simulink model "ThreeFeeder"  (R2023b)
settings: Solver=FixedStepDiscrete  StartTime=0.0  StopTime=2  RelTol=1e-3
InitFcn:
  | Frequency = 50;
  | w = 2*pi*Frequency;
  | 
  | Vnom_ph_ph = 22000;
  | Vnom = Vnom_ph_ph/sqrt(3);
  | 
  | % miles/km
  | mi2km = 1.60934;
  | % feet to km
  | ft2km = 0.0003048;
  | % microsiemens to Farads
  | ms2F = 1/2/pi/60*1e-6;
  | 
  | % Breaker
  | NOP1 = 0;
  | NOP2 = 0;
  | NOP3 = 0;
  | Fault = 0;
  | CB1 = 1;
  | CB2 = 1;
  | CB3 = 1;
undefined symbols (not defined in the file): Angle, D11, Delta, Magnitude
libraries: spsLoadFlowBusLib x24, spsThreePhasePISectionLineLib x22, spsThreePhaseVIMeasurementLib x21, spsThreePhaseSeriesRLCLoadLib x18, spsCurrentMeasurementLib x9, spsGroundLib x9, spsVoltageMeasurementLib x9, spsThreePhaseBreakerLib x6, spsThreePhaseSeriesRLCBranchLib x6, spsThreePhaseSourceLib x4, spsThreePhaseTransformerTwoWindingsLib x3, spsThreePhaseFaultLib x1
(part 1 of 2)
settings Model: Creator=liyifu  LastModifiedBy=liyifu
settings SolverCC: AlgebraicLoopSolver=TrustRegion
settings DataIOCC: ReturnWorkspaceOutputs=off
settings OptimizationCC: ReuseModelBlockBuffer=off
settings DebuggingCC: UnconnectedInputMsg=warning  UnconnectedOutputMsg=warning  UnconnectedLineMsg=warning  ArithmeticOperatorsInVariantConditions=warning
settings ModelReferenceCC: EnableRefExpFcnMdlSchedulingChecks=on
settings SFSimCC: SimUseLocalCustomCode=off  CustomCodeUndefinedFunction=UseInterfaceOnly
settings RTWCC: RTWUseLocalCustomCode=off

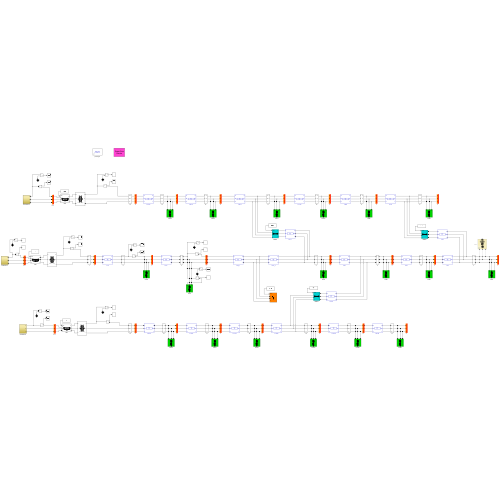
[thumbnail: Simulink's stored preview of the top-level diagram]
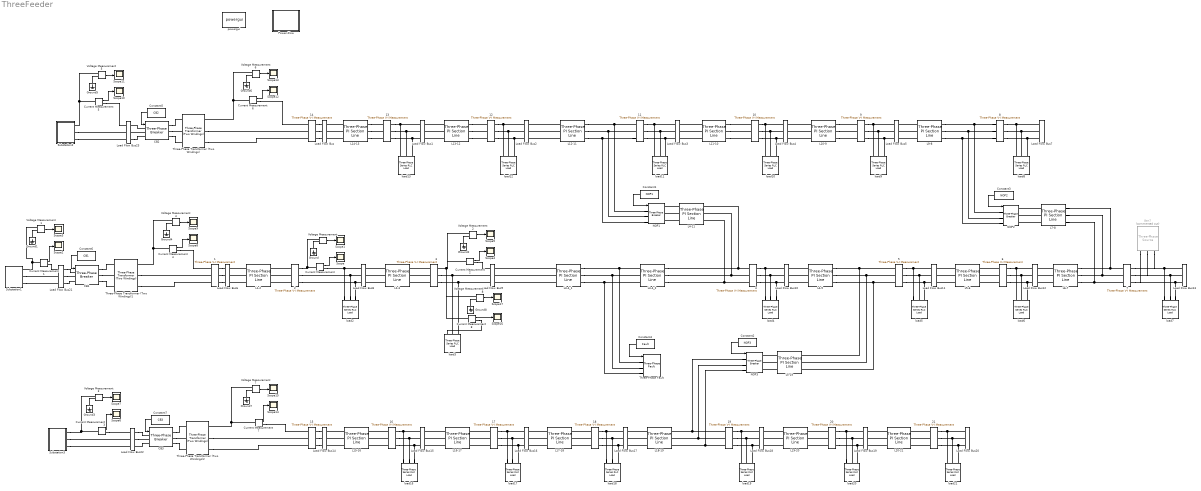
== system ThreeFeeder ==
  1 : spsThreePhaseVIMeasurementLib/Three-Phase V-I Measurement  VoltageMeasurement=phase-to-ground  SetLabelV=on  LabelV=Vabc_1  Vpu=on  VpuLL=off  CurrentMeasurement=yes  SetLabelI=on  LabelI=Iabc_1  Ipu=on  Pbase=100e6  Vbase=Vnom_ph_ph  OutputType=Magnitude-Angle  PhasorSimulation=off  PSBequivalent=0
  10 : spsThreePhaseVIMeasurementLib/Three-Phase V-I Measurement  VoltageMeasurement=phase-to-ground  SetLabelV=on  LabelV=Vabc_10  Vpu=on  VpuLL=off  CurrentMeasurement=yes  SetLabelI=on  LabelI=Iabc_10  Ipu=on  Pbase=100e6  Vbase=Vnom_ph_ph  OutputType=Magnitude-Angle  PhasorSimulation=off  PSBequivalent=0
  11 : spsThreePhaseVIMeasurementLib/Three-Phase V-I Measurement  VoltageMeasurement=phase-to-ground  SetLabelV=on  LabelV=Vabc_11  Vpu=on  VpuLL=off  CurrentMeasurement=yes  SetLabelI=on  LabelI=Iabc_11  Ipu=on  Pbase=100e6  Vbase=Vnom_ph_ph  OutputType=Magnitude-Angle  PhasorSimulation=off  PSBequivalent=0
  12 : spsThreePhaseVIMeasurementLib/Three-Phase V-I Measurement  VoltageMeasurement=phase-to-ground  SetLabelV=on  LabelV=Vabc_12  Vpu=on  VpuLL=off  CurrentMeasurement=yes  SetLabelI=on  LabelI=Iabc_12  Ipu=on  Pbase=100e6  Vbase=Vnom_ph_ph  OutputType=Magnitude-Angle  PhasorSimulation=off  PSBequivalent=0
  13 : spsThreePhaseVIMeasurementLib/Three-Phase V-I Measurement  VoltageMeasurement=phase-to-ground  SetLabelV=on  LabelV=Vabc_13  Vpu=on  VpuLL=off  CurrentMeasurement=yes  SetLabelI=on  LabelI=Iabc_13  Ipu=on  Pbase=100e6  Vbase=Vnom_ph_ph  OutputType=Magnitude-Angle  PhasorSimulation=off  PSBequivalent=0
  14 : spsThreePhaseVIMeasurementLib/Three-Phase V-I Measurement  VoltageMeasurement=phase-to-ground  SetLabelV=on  LabelV=Vabc_14  Vpu=on  VpuLL=off  CurrentMeasurement=yes  SetLabelI=on  LabelI=Iabc_14  Ipu=on  Pbase=100e6  Vbase=Vnom_ph_ph  OutputType=Magnitude-Angle  PhasorSimulation=off  PSBequivalent=0
  15 : spsThreePhaseVIMeasurementLib/Three-Phase V-I Measurement  VoltageMeasurement=phase-to-ground  SetLabelV=on  LabelV=Vabc_15  Vpu=on  VpuLL=off  CurrentMeasurement=yes  SetLabelI=on  LabelI=Iabc_15  Ipu=on  Pbase=100e6  Vbase=Vnom_ph_ph  OutputType=Magnitude-Angle  PhasorSimulation=off  PSBequivalent=0
  16 : spsThreePhaseVIMeasurementLib/Three-Phase V-I Measurement  VoltageMeasurement=phase-to-ground  SetLabelV=on  LabelV=Vabc_16  Vpu=on  VpuLL=off  CurrentMeasurement=yes  SetLabelI=on  LabelI=Iabc_16  Ipu=on  Pbase=100e6  Vbase=Vnom_ph_ph  OutputType=Magnitude-Angle  PhasorSimulation=off  PSBequivalent=0
  17 : spsThreePhaseVIMeasurementLib/Three-Phase V-I Measurement  VoltageMeasurement=phase-to-ground  SetLabelV=on  LabelV=Vabc_17  Vpu=on  VpuLL=off  CurrentMeasurement=yes  SetLabelI=on  LabelI=Iabc_17  Ipu=on  Pbase=100e6  Vbase=Vnom_ph_ph  OutputType=Magnitude-Angle  PhasorSimulation=off  PSBequivalent=0
  18 : spsThreePhaseVIMeasurementLib/Three-Phase V-I Measurement  VoltageMeasurement=phase-to-ground  SetLabelV=on  LabelV=Vabc_18  Vpu=on  VpuLL=off  CurrentMeasurement=yes  SetLabelI=on  LabelI=Iabc_18  Ipu=on  Pbase=100e6  Vbase=Vnom_ph_ph  OutputType=Magnitude-Angle  PhasorSimulation=off  PSBequivalent=0
  19 : spsThreePhaseVIMeasurementLib/Three-Phase V-I Measurement  VoltageMeasurement=phase-to-ground  SetLabelV=on  LabelV=Vabc_19  Vpu=on  VpuLL=off  CurrentMeasurement=yes  SetLabelI=on  LabelI=Iabc_19  Ipu=on  Pbase=100e6  Vbase=Vnom_ph_ph  OutputType=Magnitude-Angle  PhasorSimulation=off  PSBequivalent=0
  2 : spsThreePhaseVIMeasurementLib/Three-Phase V-I Measurement  VoltageMeasurement=phase-to-ground  SetLabelV=on  LabelV=Vabc_2  Vpu=on  VpuLL=off  CurrentMeasurement=yes  SetLabelI=on  LabelI=Iabc_2  Ipu=on  Pbase=100e6  Vbase=Vnom_ph_ph  OutputType=Magnitude-Angle  PhasorSimulation=off  PSBequivalent=0
  20 : spsThreePhaseVIMeasurementLib/Three-Phase V-I Measurement  VoltageMeasurement=phase-to-ground  SetLabelV=on  LabelV=Vabc_20  Vpu=on  VpuLL=off  CurrentMeasurement=yes  SetLabelI=on  LabelI=Iabc_20  Ipu=on  Pbase=100e6  Vbase=Vnom_ph_ph  OutputType=Magnitude-Angle  PhasorSimulation=off  PSBequivalent=0
  21 : spsThreePhaseVIMeasurementLib/Three-Phase V-I Measurement  VoltageMeasurement=phase-to-ground  SetLabelV=on  LabelV=Vabc_21  Vpu=on  VpuLL=off  CurrentMeasurement=yes  SetLabelI=on  LabelI=Iabc_21  Ipu=on  Pbase=100e6  Vbase=Vnom_ph_ph  OutputType=Magnitude-Angle  PhasorSimulation=off  PSBequivalent=0
  3 : spsThreePhaseVIMeasurementLib/Three-Phase V-I Measurement  VoltageMeasurement=phase-to-ground  SetLabelV=on  LabelV=Vabc_3  Vpu=on  VpuLL=off  CurrentMeasurement=yes  SetLabelI=on  LabelI=Iabc_3  Ipu=on  Pbase=100e6  Vbase=Vnom_ph_ph  OutputType=Magnitude-Angle  PhasorSimulation=off  PSBequivalent=0
  4 : spsThreePhaseVIMeasurementLib/Three-Phase V-I Measurement  VoltageMeasurement=phase-to-ground  SetLabelV=on  LabelV=Vabc_4  Vpu=on  VpuLL=off  CurrentMeasurement=yes  SetLabelI=on  LabelI=Iabc_4  Ipu=on  Pbase=100e6  Vbase=Vnom_ph_ph  OutputType=Magnitude-Angle  PhasorSimulation=off  PSBequivalent=0
  5 : spsThreePhaseVIMeasurementLib/Three-Phase V-I Measurement  VoltageMeasurement=phase-to-ground  SetLabelV=on  LabelV=Vabc_5  Vpu=on  VpuLL=off  CurrentMeasurement=yes  SetLabelI=on  LabelI=Iabc_5  Ipu=on  Pbase=100e6  Vbase=Vnom_ph_ph  OutputType=Magnitude-Angle  PhasorSimulation=off  PSBequivalent=0
  6 : spsThreePhaseVIMeasurementLib/Three-Phase V-I Measurement  VoltageMeasurement=phase-to-ground  SetLabelV=on  LabelV=Vabc_6  Vpu=on  VpuLL=off  CurrentMeasurement=yes  SetLabelI=on  LabelI=Iabc_6  Ipu=on  Pbase=100e6  Vbase=Vnom_ph_ph  OutputType=Magnitude-Angle  PhasorSimulation=off  PSBequivalent=0
  7 : spsThreePhaseVIMeasurementLib/Three-Phase V-I Measurement  VoltageMeasurement=phase-to-ground  SetLabelV=on  LabelV=Vabc_7  Vpu=on  VpuLL=off  CurrentMeasurement=yes  SetLabelI=on  LabelI=Iabc_7  Ipu=on  Pbase=100e6  Vbase=Vnom_ph_ph  OutputType=Magnitude-Angle  PhasorSimulation=off  PSBequivalent=0
  8 : spsThreePhaseVIMeasurementLib/Three-Phase V-I Measurement  VoltageMeasurement=phase-to-ground  SetLabelV=on  LabelV=Vabc_8  Vpu=on  VpuLL=off  CurrentMeasurement=yes  SetLabelI=on  LabelI=Iabc_8  Ipu=on  Pbase=100e6  Vbase=Vnom_ph_ph  OutputType=Magnitude-Angle  PhasorSimulation=off  PSBequivalent=0
  9 : spsThreePhaseVIMeasurementLib/Three-Phase V-I Measurement  VoltageMeasurement=phase-to-ground  SetLabelV=on  LabelV=Vabc_9  Vpu=on  VpuLL=off  CurrentMeasurement=yes  SetLabelI=on  LabelI=Iabc_9  Ipu=on  Pbase=100e6  Vbase=Vnom_ph_ph  OutputType=Magnitude-Angle  PhasorSimulation=off  PSBequivalent=0
  CB1 : spsThreePhaseBreakerLib/Three-Phase Breaker  InitialState=closed  SwitchA=on  SwitchB=on  SwitchC=on  SwitchTimes="[1/60  5/60]"  External=on  BreakerResistance=0.01  SnubberResistance=1e6  SnubberCapacitance=inf  Measurements=None
  CB2 : spsThreePhaseBreakerLib/Three-Phase Breaker  InitialState=closed  SwitchA=on  SwitchB=on  SwitchC=on  SwitchTimes="[1/60  5/60]"  External=on  BreakerResistance=0.01  SnubberResistance=1e6  SnubberCapacitance=inf  Measurements=None
  CB3 : spsThreePhaseBreakerLib/Three-Phase Breaker  InitialState=closed  SwitchA=on  SwitchB=on  SwitchC=on  SwitchTimes="[1/60  5/60]"  External=on  BreakerResistance=0.01  SnubberResistance=1e6  SnubberCapacitance=inf  Measurements=None
  Constant1 : Constant  Value=NOP1
  Constant2 : Constant  Value=NOP3
  Constant3 : Constant  Value=NOP2
  Constant4 : Constant  Value=Fault
  Constant5 : Constant  Value=CB2
  Constant6 : Constant  Value=CB1
  Constant7 : Constant  Value=CB3
  Current Measurement{,1..8} (9 alike) : spsCurrentMeasurementLib/Current Measurement  PhasorSimulation=off  OutputType=Magnitude  PSBequivalent=0
  Gen7 : spsThreePhaseSourceLib/Three-Phase Source  Commented=on  InternalConnection=Yg  VoltagePhases=off  Voltage=22e3  PhaseAngle=0  Voltage_phases=[1 1 1]*(115e3)/sqrt(3)  PhaseAngles_phases=[0 -120 +120]  Frequency=60  NonIdealSource=on  SpecifyImpedance=off  Resistance=1  Inductance=1e-6  ShortCircuitLevel=Apparent_power_gen1  BaseVoltage=Vnom_ph_ph  XRratio=8  BusType=PQ  Pref=29.05e6  Qref=3.10e6  Prefabc=[10e3, 10e3, 10e3]  Qrefabc=[0, 0, 0]  Qmin=-inf  Qmax=inf
  Ground{,1..8} (9 alike) : spsGroundLib/Ground  LConnTagsString=a
  L1-2 : spsThreePhasePISectionLineLib/Three-Phase PI Section Line  LConnTagsString=a|b|c  RConnTagsString=A|B|C  Length=1  Frequency=60  Resistances=[0.000845366 0.3864]  Inductances="[0.000284806/w  4.1264e-3]"  Capacitances=[0.057272218/w 7.751e-9]
  L10-9 : spsThreePhasePISectionLineLib/Three-Phase PI Section Line  LConnTagsString=a|b|c  RConnTagsString=A|B|C  Length=1  Frequency=60  Resistances=[5.29711e-05 0.3864]  Inductances="[2.71261e-05/w  4.1264e-3]"  Capacitances=[0.005556479/w 7.751e-9]
  L11-10 : spsThreePhasePISectionLineLib/Three-Phase PI Section Line  LConnTagsString=a|b|c  RConnTagsString=A|B|C  Length=1  Frequency=60  Resistances=[8.33801e-05 0.3864]  Inductances="[3.95703e-05/w  4.1264e-3]"  Capacitances=[0.008970369/w 7.751e-9]
  L12-11 : spsThreePhasePISectionLineLib/Three-Phase PI Section Line  LConnTagsString=a|b|c  RConnTagsString=A|B|C  Length=1  Frequency=60  Resistances=[0.000186264 0.3864]  Inductances="[8.83967e-05/w  4.1264e-3]"  Capacitances=[0.020039071/w 7.751e-9]
  L13-12 : spsThreePhasePISectionLineLib/Three-Phase PI Section Line  LConnTagsString=a|b|c  RConnTagsString=A|B|C  Length=1  Frequency=60  Resistances=[0.000650678 0.3864]  Inductances="[0.000465415/w  4.1264e-3]"  Capacitances=[0.138669141/w 7.751e-9]
  L14-13 : spsThreePhasePISectionLineLib/Three-Phase PI Section Line  LConnTagsString=a|b|c  RConnTagsString=A|B|C  Length=1  Frequency=60  Resistances=[0.000845366 0.3864]  Inductances="[0.000284806/w  4.1264e-3]"  Capacitances=[0.057272218/w 7.751e-9]
  L15-16 : spsThreePhasePISectionLineLib/Three-Phase PI Section Line  LConnTagsString=a|b|c  RConnTagsString=A|B|C  Length=1  Frequency=60  Resistances=[0.000394176 0.3864]  Inductances="[0.000135417/w  4.1264e-3]"  Capacitances=[0.026794351/w 7.751e-9]
  L16-17 : spsThreePhasePISectionLineLib/Three-Phase PI Section Line  LConnTagsString=a|b|c  RConnTagsString=A|B|C  Length=1  Frequency=60  Resistances=[0.000394176 0.3864]  Inductances="[0.000135417/w  4.1264e-3]"  Capacitances=[0.026794351/w 7.751e-9]
  L17-18 : spsThreePhasePISectionLineLib/Three-Phase PI Section Line  LConnTagsString=a|b|c  RConnTagsString=A|B|C  Length=1  Frequency=60  Resistances=[0.000394176 0.3864]  Inductances="[0.000135417/w  4.1264e-3]"  Capacitances=[0.026794351/w 7.751e-9]
  L18-19 : spsThreePhasePISectionLineLib/Three-Phase PI Section Line  LConnTagsString=a|b|c  RConnTagsString=A|B|C  Length=1  Frequency=60  Resistances=[0.000394176 0.3864]  Inductances="[0.000135417/w  4.1264e-3]"  Capacitances=[0.026794351/w 7.751e-9]
  L19-20 : spsThreePhasePISectionLineLib/Three-Phase PI Section Line  LConnTagsString=a|b|c  RConnTagsString=A|B|C  Length=1  Frequency=60  Resistances=[0.000394176 0.3864]  Inductances="[0.000135417/w  4.1264e-3]"  Capacitances=[0.026794351/w 7.751e-9]
  L2-3 : spsThreePhasePISectionLineLib/Three-Phase PI Section Line  LConnTagsString=a|b|c  RConnTagsString=A|B|C  Length=1  Frequency=60  Resistances=[0.000845366 0.3864]  Inductances="[0.000284806/w  4.1264e-3]"  Capacitances=[0.057272218/w 7.751e-9]
  L20-21 : spsThreePhasePISectionLineLib/Three-Phase PI Section Line  LConnTagsString=a|b|c  RConnTagsString=A|B|C  Length=1  Frequency=60  Resistances=[0.000394176 0.3864]  Inductances="[0.000135417/w  4.1264e-3]"  Capacitances=[0.026794351/w 7.751e-9]
  L3-4_1 : spsThreePhasePISectionLineLib/Three-Phase PI Section Line  LConnTagsString=a|b|c  RConnTagsString=A|B|C  Length=0.5  Frequency=60  Resistances=[0.000845366 0.3864]  Inductances="[0.000284806/w  4.1264e-3]"  Capacitances=[0.057272218/w 7.751e-9]
  L3-4_2 : spsThreePhasePISectionLineLib/Three-Phase PI Section Line  LConnTagsString=a|b|c  RConnTagsString=A|B|C  Length=0.5  Frequency=60  Resistances=[0.000845366 0.3864]  Inductances="[0.000284806/w  4.1264e-3]"  Capacitances=[0.057272218/w 7.751e-9]
  L4-11 : spsThreePhasePISectionLineLib/Three-Phase PI Section Line  LConnTagsString=a|b|c  RConnTagsString=A|B|C  Length=1  Frequency=60  Resistances=[8.33801e-05 0.3864]  Inductances="[3.95703e-05/w  4.1264e-3]"  Capacitances=[0.008970369 7.751e-9]
  L4-5 : spsThreePhasePISectionLineLib/Three-Phase PI Section Line  LConnTagsString=a|b|c  RConnTagsString=A|B|C  Length=1  Frequency=60  Resistances=[3.90909e-05 0.3864]  Inductances="[2.39876e-05/w  4.1264e-3]"  Capacitances=[0.006538279/w 7.751e-9]
  L5-19 : spsThreePhasePISectionLineLib/Three-Phase PI Section Line  LConnTagsString=a|b|c  RConnTagsString=A|B|C  Length=1  Frequency=60  Resistances=[0.000394176 0.3864]  Inductances="[0.000135417/w  4.1264e-3]"  Capacitances=[0.026794351/w 7.751e-9]
  L5-6 : spsThreePhasePISectionLineLib/Three-Phase PI Section Line  LConnTagsString=a|b|c  RConnTagsString=A|B|C  Length=1  Frequency=60  Resistances=[0.001065536 0.3864]  Inductances="[0.00075818/w  4.1264e-3]"  Capacitances=[0.225289616/w 7.751e-9]
  L6-7 : spsThreePhasePISectionLineLib/Three-Phase PI Section Line  LConnTagsString=a|b|c  RConnTagsString=A|B|C  Length=1  Frequency=60  Resistances=[0.000394176 0.3864]  Inductances="[0.000135417/w  4.1264e-3]"  Capacitances=[0.026794351/w 7.751e-9]
  L7-8 : spsThreePhasePISectionLineLib/Three-Phase PI Section Line  LConnTagsString=a|b|c  RConnTagsString=A|B|C  Length=1  Frequency=60  Resistances=[0.000394176 0.3864]  Inductances="[0.000135417/w  4.1264e-3]"  Capacitances=[0.026794351/w 7.751e-9]
  L9-8 : spsThreePhasePISectionLineLib/Three-Phase PI Section Line  LConnTagsString=a|b|c  RConnTagsString=A|B|C  Length=1  Frequency=60  Resistances=[4.96363e-05 0.3864]  Inductances="[2.64194e-05/w  4.1264e-3]"  Capacitances=[0.005739856/w 7.751e-9]
  Load Flow Bus : spsLoadFlowBusLib/Load Flow Bus  LConnTagsString=a|b|c  RConnTagsString=a|b|c  Phases=ABC  Connectors=on both sides  ID=14  Vbase=Vnom  Vref="[1  1  1]"  Vangle="[0  -120  120]"  VLF=1  VLFb=1  VLFc=1  angleLF=0  angleLFb=0  angleLFc=0
      settings: AttributesFormatString=%<ID>
  Load Flow Bus1 : spsLoadFlowBusLib/Load Flow Bus  LConnTagsString=a|b|c  RConnTagsString=a|b|c  Phases=ABC  Connectors=on both sides  ID=13  Vbase=Vnom  Vref=[1 1 1]  Vangle="[0  -120  120]"  VLF=1  VLFb=1  VLFc=1  angleLF=0  angleLFb=0  angleLFc=0
      settings: AttributesFormatString=%<ID>
  Load Flow Bus10 : spsLoadFlowBusLib/Load Flow Bus  LConnTagsString=a|b|c  RConnTagsString=a|b|c  Phases=ABC  Connectors=on both sides  ID=4  Vbase=Vnom  Vref=[1 1 1]  Vangle="[0  -120  120]"  VLF=1  VLFb=1  VLFc=1  angleLF=0  angleLFb=0  angleLFc=0
      settings: AttributesFormatString=%<ID>
  Load Flow Bus11 : spsLoadFlowBusLib/Load Flow Bus  LConnTagsString=a|b|c  RConnTagsString=a|b|c  Phases=ABC  Connectors=on both sides  ID=5  Vbase=Vnom  Vref=[1 1 1]  Vangle="[0  -120  120]"  VLF=1  VLFb=1  VLFc=1  angleLF=0  angleLFb=0  angleLFc=0
      settings: AttributesFormatString=%<ID>
  Load Flow Bus12 : spsLoadFlowBusLib/Load Flow Bus  LConnTagsString=a|b|c  RConnTagsString=a|b|c  Phases=ABC  Connectors=on both sides  ID=6  Vbase=Vnom  Vref=[1 1 1]  Vangle="[0  -120  120]"  VLF=1  VLFb=1  VLFc=1  angleLF=0  angleLFb=0  angleLFc=0
      settings: AttributesFormatString=%<ID>
  Load Flow Bus13 : spsLoadFlowBusLib/Load Flow Bus  LConnTagsString=a|b|c  Phases=ABC  Connectors=on one side  ID=7  Vbase=Vnom  Vref=[1 1 1]  Vangle="[0  -120  120]"  VLF=1  VLFb=1  VLFc=1  angleLF=0  angleLFb=0  angleLFc=0
      settings: AttributesFormatString=%<ID>
  Load Flow Bus14 : spsLoadFlowBusLib/Load Flow Bus  LConnTagsString=a|b|c  RConnTagsString=a|b|c  Phases=ABC  Connectors=on both sides  ID=15  Vbase=Vnom  Vref="[1  1  1]"  Vangle="[0  -120  120]"  VLF=1  VLFb=1  VLFc=1  angleLF=0  angleLFb=0  angleLFc=0
      settings: AttributesFormatString=%<ID>
  Load Flow Bus15 : spsLoadFlowBusLib/Load Flow Bus  LConnTagsString=a|b|c  RConnTagsString=a|b|c  Phases=ABC  Connectors=on both sides  ID=16  Vbase=Vnom  Vref=[1 1 1]  Vangle="[0  -120  120]"  VLF=1  VLFb=1  VLFc=1  angleLF=0  angleLFb=0  angleLFc=0
      settings: AttributesFormatString=%<ID>
  Load Flow Bus16 : spsLoadFlowBusLib/Load Flow Bus  LConnTagsString=a|b|c  RConnTagsString=a|b|c  Phases=ABC  Connectors=on both sides  ID=17  Vbase=Vnom  Vref=[1 1 1]  Vangle="[0  -120  120]"  VLF=1  VLFb=1  VLFc=1  angleLF=0  angleLFb=0  angleLFc=0
      settings: AttributesFormatString=%<ID>
  Load Flow Bus17 : spsLoadFlowBusLib/Load Flow Bus  LConnTagsString=a|b|c  RConnTagsString=a|b|c  Phases=ABC  Connectors=on both sides  ID=18  Vbase=Vnom  Vref=[1 1 1]  Vangle="[0  -120  120]"  VLF=1  VLFb=1  VLFc=1  angleLF=0  angleLFb=0  angleLFc=0
      settings: AttributesFormatString=%<ID>
  Load Flow Bus18 : spsLoadFlowBusLib/Load Flow Bus  LConnTagsString=a|b|c  RConnTagsString=a|b|c  Phases=ABC  Connectors=on both sides  ID=19  Vbase=Vnom  Vref=[1 1 1]  Vangle="[0  -120  120]"  VLF=1  VLFb=1  VLFc=1  angleLF=0  angleLFb=0  angleLFc=0
      settings: AttributesFormatString=%<ID>
  Load Flow Bus19 : spsLoadFlowBusLib/Load Flow Bus  LConnTagsString=a|b|c  RConnTagsString=a|b|c  Phases=ABC  Connectors=on both sides  ID=20  Vbase=Vnom  Vref=[1 1 1]  Vangle="[0  -120  120]"  VLF=1  VLFb=1  VLFc=1  angleLF=0  angleLFb=0  angleLFc=0
      settings: AttributesFormatString=%<ID>
  Load Flow Bus2 : spsLoadFlowBusLib/Load Flow Bus  LConnTagsString=a|b|c  RConnTagsString=a|b|c  Phases=ABC  Connectors=on both sides  ID=12  Vbase=Vnom  Vref=[1 1 1]  Vangle="[0  -120  120]"  VLF=1  VLFb=1  VLFc=1  angleLF=0  angleLFb=0  angleLFc=0
      settings: AttributesFormatString=%<ID>
  Load Flow Bus20 : spsLoadFlowBusLib/Load Flow Bus  LConnTagsString=a|b|c  Phases=ABC  Connectors=on one side  ID=21  Vbase=Vnom  Vref=[1 1 1]  Vangle="[0  -120  120]"  VLF=1  VLFb=1  VLFc=1  angleLF=0  angleLFb=0  angleLFc=0
      settings: AttributesFormatString=%<ID>
  Load Flow Bus21 : spsLoadFlowBusLib/Load Flow Bus  LConnTagsString=a|b|c  RConnTagsString=a|b|c  Phases=ABC  Connectors=on both sides  ID=HV1  Vbase=Vnom  Vref="[1  1  1]"  Vangle="[0  -120  120]"  VLF=1  VLFb=1  VLFc=1  angleLF=0  angleLFb=0  angleLFc=0
      settings: AttributesFormatString=%<ID>
  Load Flow Bus22 : spsLoadFlowBusLib/Load Flow Bus  LConnTagsString=a|b|c  RConnTagsString=a|b|c  Phases=ABC  Connectors=on both sides  ID=HV3  Vbase=Vnom  Vref="[1  1  1]"  Vangle="[0  -120  120]"  VLF=1  VLFb=1  VLFc=1  angleLF=0  angleLFb=0  angleLFc=0
      settings: AttributesFormatString=%<ID>
  Load Flow Bus23 : spsLoadFlowBusLib/Load Flow Bus  LConnTagsString=a|b|c  RConnTagsString=a|b|c  Phases=ABC  Connectors=on both sides  ID=HV2  Vbase=Vnom  Vref="[1  1  1]"  Vangle="[0  -120  120]"  VLF=1  VLFb=1  VLFc=1  angleLF=0  angleLFb=0  angleLFc=0
      settings: AttributesFormatString=%<ID>
  Load Flow Bus3 : spsLoadFlowBusLib/Load Flow Bus  LConnTagsString=a|b|c  RConnTagsString=a|b|c  Phases=ABC  Connectors=on both sides  ID=11  Vbase=Vnom  Vref=[1 1 1]  Vangle="[0  -120  120]"  VLF=1  VLFb=1  VLFc=1  angleLF=0  angleLFb=0  angleLFc=0
      settings: AttributesFormatString=%<ID>
  Load Flow Bus4 : spsLoadFlowBusLib/Load Flow Bus  LConnTagsString=a|b|c  RConnTagsString=a|b|c  Phases=ABC  Connectors=on both sides  ID=10  Vbase=Vnom  Vref=[1 1 1]  Vangle="[0  -120  120]"  VLF=1  VLFb=1  VLFc=1  angleLF=0  angleLFb=0  angleLFc=0
      settings: AttributesFormatString=%<ID>
  Load Flow Bus5 : spsLoadFlowBusLib/Load Flow Bus  LConnTagsString=a|b|c  RConnTagsString=a|b|c  Phases=ABC  Connectors=on both sides  ID=9  Vbase=Vnom  Vref=[1 1 1]  Vangle="[0  -120  120]"  VLF=1  VLFb=1  VLFc=1  angleLF=0  angleLFb=0  angleLFc=0
      settings: AttributesFormatString=%<ID>
  Load Flow Bus6 : spsLoadFlowBusLib/Load Flow Bus  LConnTagsString=a|b|c  RConnTagsString=a|b|c  Phases=ABC  Connectors=on both sides  ID=1  Vbase=Vnom  Vref="[1  1  1]"  Vangle="[0  -120  120]"  VLF=1  VLFb=1  VLFc=1  angleLF=0  angleLFb=0  angleLFc=0
      settings: AttributesFormatString=%<ID>
  Load Flow Bus7 : spsLoadFlowBusLib/Load Flow Bus  LConnTagsString=a|b|c  Phases=ABC  Connectors=on one side  ID=8  Vbase=Vnom  Vref=[1 1 1]  Vangle="[0  -120  120]"  VLF=1  VLFb=1  VLFc=1  angleLF=0  angleLFb=0  angleLFc=0
      settings: AttributesFormatString=%<ID>
  Load Flow Bus8 : spsLoadFlowBusLib/Load Flow Bus  LConnTagsString=a|b|c  RConnTagsString=a|b|c  Phases=ABC  Connectors=on both sides  ID=2  Vbase=Vnom  Vref=[1 1 1]  Vangle="[0  -120  120]"  VLF=1  VLFb=1  VLFc=1  angleLF=0  angleLFb=0  angleLFc=0
      settings: AttributesFormatString=%<ID>
  Load Flow Bus9 : spsLoadFlowBusLib/Load Flow Bus  LConnTagsString=a|b|c  RConnTagsString=a|b|c  Phases=ABC  Connectors=on both sides  ID=3  Vbase=Vnom  Vref=[1 1 1]  Vangle="[0  -120  120]"  VLF=1  VLFb=1  VLFc=1  angleLF=0  angleLFb=0  angleLFc=0
      settings: AttributesFormatString=%<ID>
  NOP1 : spsThreePhaseBreakerLib/Three-Phase Breaker  InitialState=closed  SwitchA=on  SwitchB=on  SwitchC=on  SwitchTimes=[0.5 ]  External=on  BreakerResistance=0.0001  SnubberResistance=inf  SnubberCapacitance=0  Measurements=None
  NOP2 : spsThreePhaseBreakerLib/Three-Phase Breaker  InitialState=closed  SwitchA=on  SwitchB=on  SwitchC=on  SwitchTimes=[0.5 ]  External=on  BreakerResistance=0.0001  SnubberResistance=inf  SnubberCapacitance=0  Measurements=None
  NOP3 : spsThreePhaseBreakerLib/Three-Phase Breaker  InitialState=closed  SwitchA=on  SwitchB=on  SwitchC=on  SwitchTimes=[0.5 ]  External=on  BreakerResistance=0.0001  SnubberResistance=inf  SnubberCapacitance=0  Measurements=None
  Power-Flow : Subsystem
      mask Display: disp('Power-Flow\nResults')
  Scope{,1..17} (18 alike) : Scope
  Substation1 : Subsystem
  Substation2 : Subsystem
  Substation3 : Subsystem
  Three-Phase Transformer (Two Windings) : spsThreePhaseTransformerTwoWindingsLib/Three-Phase Transformer (Two Windings)  Winding1Connection=Delta (D11)  Winding2Connection=Yg  CoreType=Three single-phase transformers  SetSaturation=off  Hysteresis=off  DataFile='hysteresis'  SetInitialFlux=off  Measurements=None  UNITS=pu  NominalPower=[300e6, Frequency]  Winding1=[115000, 0.01, 0.01]  Winding2=[22000, 0.01, 0.01]  Rm=500  Lm=500  L0=0.5  Saturation=[0 0;0.0024001 1;1 1.2667]  InitialFluxes=[ 0.8 , -0.8 , 0.7 ]  BreakLoop=off  DiscreteSolver=Trapezoidal iterative  DataType=off  TransfoNumber=1
  Three-Phase Transformer (Two Windings)1 : spsThreePhaseTransformerTwoWindingsLib/Three-Phase Transformer (Two Windings)  Winding1Connection=Delta (D11)  Winding2Connection=Yg  CoreType=Three single-phase transformers  SetSaturation=off  Hysteresis=off  DataFile='hysteresis'  SetInitialFlux=off  Measurements=None  UNITS=pu  NominalPower=[300e6, Frequency]  Winding1=[115000, 0.04, 0.02]  Winding2=[22000, 0.04, 0.02]  Rm=500  Lm=500  L0=0.5  Saturation=[0 0;0.0024001 1;1 1.2667]  InitialFluxes=[ 0.8 , -0.8 , 0.7 ]  BreakLoop=off  DiscreteSolver=Trapezoidal iterative  DataType=off  TransfoNumber=1
  Three-Phase Transformer (Two Windings)2 : spsThreePhaseTransformerTwoWindingsLib/Three-Phase Transformer (Two Windings)  Winding1Connection=Delta (D11)  Winding2Connection=Yg  CoreType=Three single-phase transformers  SetSaturation=off  Hysteresis=off  DataFile='hysteresis'  SetInitialFlux=off  Measurements=None  UNITS=pu  NominalPower=[300e6, Frequency]  Winding1=[120000, 0.01, 0.01]  Winding2=[22000, 0.01, 0.01]  Rm=500  Lm=500  L0=0.5  Saturation=[0 0;0.0025044 0.95833;1.0435 1.2139]  InitialFluxes=[ 0.8 , -0.8 , 0.7 ]  BreakLoop=off  DiscreteSolver=Trapezoidal iterative  DataType=off  TransfoNumber=1
  Three-Phase Fault : spsThreePhaseFaultLib/Three-Phase Fault  InitialStates=0  FaultA=on  FaultB=off  FaultC=off  GroundFault=on  SwitchTimes="[1/60  5/60]"  External=on  SwitchStatus=NaN  FaultResistance=0.001  GroundResistance=0.01  SnubberResistance=1e6  SnubberCapacitance=inf  Measurements=None
  Voltage Measurement{,1..8} (9 alike) : spsVoltageMeasurementLib/Voltage Measurement  PhasorSimulation=off  OutputType=Magnitude  PSBequivalent=0
  load10 : spsThreePhaseSeriesRLCLoadLib/Three-Phase Series RLC Load  LConnTagsString=A|B|C  Configuration=Y (grounded)  NominalVoltage=Vnom_ph_ph  Vabc=[1e3 1e3 1e3]  Vabcp=[1e3 1e3 1e3]  NominalFrequency=60  UnbalancedPower=off  ActivePower=190.3e6  InductivePower=81.38e6  CapacitivePower=0  Pabc=[10e3 9e3 11e3]  QLabc=[100 90 110]  QCabc=[100 90 110]  Pabcp=[10e3 9e3 11e3]  QLabcp=[100 90 110]  QCabcp=[100 90 110]  Measurements=None  LoadType=constant Z
  load11 : spsThreePhaseSeriesRLCLoadLib/Three-Phase Series RLC Load  LConnTagsString=A|B|C  Configuration=Y (grounded)  NominalVoltage=Vnom_ph_ph  Vabc=[1e3 1e3 1e3]  Vabcp=[1e3 1e3 1e3]  NominalFrequency=60  UnbalancedPower=off  ActivePower=27.46e6  InductivePower=5.35e6  CapacitivePower=0  Pabc=[10e3 9e3 11e3]  QLabc=[100 90 110]  QCabc=[100 90 110]  Pabcp=[10e3 9e3 11e3]  QLabcp=[100 90 110]  QCabcp=[100 90 110]  Measurements=None  LoadType=constant Z
  load12 : spsThreePhaseSeriesRLCLoadLib/Three-Phase Series RLC Load  LConnTagsString=A|B|C  Configuration=Y (grounded)  NominalVoltage=Vnom_ph_ph  Vabc=[1e3 1e3 1e3]  Vabcp=[1e3 1e3 1e3]  NominalFrequency=60  UnbalancedPower=off  ActivePower=32.82e6  InductivePower=5.02e6  CapacitivePower=0  Pabc=[10e3 9e3 11e3]  QLabc=[100 90 110]  QCabc=[100 90 110]  Pabcp=[10e3 9e3 11e3]  QLabcp=[100 90 110]  QCabcp=[100 90 110]  Measurements=None  LoadType=constant Z
  load{2..3,13,16,20..21} (6 alike) : spsThreePhaseSeriesRLCLoadLib/Three-Phase Series RLC Load  LConnTagsString=A|B|C  Configuration=Y (grounded)  NominalVoltage=Vnom_ph_ph  Vabc=[1e3 1e3 1e3]  Vabcp=[1e3 1e3 1e3]  NominalFrequency=60  UnbalancedPower=off  ActivePower=38.59e6  InductivePower=5.42e6  CapacitivePower=0  Pabc=[10e3 9e3 11e3]  QLabc=[100 90 110]  QCabc=[100 90 110]  Pabcp=[10e3 9e3 11e3]  QLabcp=[100 90 110]  QCabcp=[100 90 110]  Measurements=None  LoadType=constant Z
  load17 : spsThreePhaseSeriesRLCLoadLib/Three-Phase Series RLC Load  LConnTagsString=A|B|C  Configuration=Y (grounded)  NominalVoltage=Vnom_ph_ph  Vabc=[1e3 1e3 1e3]  Vabcp=[1e3 1e3 1e3]  NominalFrequency=60  UnbalancedPower=off  ActivePower=38.15e6  InductivePower=5.47e6  CapacitivePower=0  Pabc=[10e3 9e3 11e3]  QLabc=[100 90 110]  QCabc=[100 90 110]  Pabcp=[10e3 9e3 11e3]  QLabcp=[100 90 110]  QCabcp=[100 90 110]  Measurements=None  LoadType=constant Z
  load18 : spsThreePhaseSeriesRLCLoadLib/Three-Phase Series RLC Load  LConnTagsString=A|B|C  Configuration=Y (grounded)  NominalVoltage=Vnom_ph_ph  Vabc=[1e3 1e3 1e3]  Vabcp=[1e3 1e3 1e3]  NominalFrequency=60  UnbalancedPower=off  ActivePower=27.46e6  InductivePower=5.35e6  CapacitivePower=0  Pabc=[10e3 9e3 11e3]  QLabc=[100 90 110]  QCabc=[100 90 110]  Pabcp=[10e3 9e3 11e3]  QLabcp=[100 90 110]  QCabcp=[100 90 110]  Measurements=None  LoadType=constant Z
  load19 : spsThreePhaseSeriesRLCLoadLib/Three-Phase Series RLC Load  LConnTagsString=A|B|C  Configuration=Y (grounded)  NominalVoltage=Vnom_ph_ph  Vabc=[1e3 1e3 1e3]  Vabcp=[1e3 1e3 1e3]  NominalFrequency=60  UnbalancedPower=off  ActivePower=32.82e6  InductivePower=5.02e6  CapacitivePower=0  Pabc=[10e3 9e3 11e3]  QLabc=[100 90 110]  QCabc=[100 90 110]  Pabcp=[10e3 9e3 11e3]  QLabcp=[100 90 110]  QCabcp=[100 90 110]  Measurements=None  LoadType=constant Z
  load4 : spsThreePhaseSeriesRLCLoadLib/Three-Phase Series RLC Load  LConnTagsString=A|B|C  Configuration=Y (grounded)  NominalVoltage=Vnom_ph_ph  Vabc=[1e3 1e3 1e3]  Vabcp=[1e3 1e3 1e3]  NominalFrequency=60  UnbalancedPower=off  ActivePower=34.95e6  InductivePower=5.11e6  CapacitivePower=0  Pabc=[10e3 9e3 11e3]  QLabc=[100 90 110]  QCabc=[100 90 110]  Pabcp=[10e3 9e3 11e3]  QLabcp=[100 90 110]  QCabcp=[100 90 110]  Measurements=None  LoadType=constant Z
  load5 : spsThreePhaseSeriesRLCLoadLib/Three-Phase Series RLC Load  LConnTagsString=A|B|C  Configuration=Y (grounded)  NominalVoltage=Vnom_ph_ph  Vabc=[1e3 1e3 1e3]  Vabcp=[1e3 1e3 1e3]  NominalFrequency=60  UnbalancedPower=off  ActivePower=38.15e6  InductivePower=5.47e6  CapacitivePower=0  Pabc=[10e3 9e3 11e3]  QLabc=[100 90 110]  QCabc=[100 90 110]  Pabcp=[10e3 9e3 11e3]  QLabcp=[100 90 110]  QCabcp=[100 90 110]  Measurements=None  LoadType=constant Z
  load6 : spsThreePhaseSeriesRLCLoadLib/Three-Phase Series RLC Load  LConnTagsString=A|B|C  Configuration=Y (grounded)  NominalVoltage=Vnom_ph_ph  Vabc=[1e3 1e3 1e3]  Vabcp=[1e3 1e3 1e3]  NominalFrequency=60  UnbalancedPower=off  ActivePower=30.05e6  InductivePower=5.19e6  CapacitivePower=0  Pabc=[10e3 9e3 11e3]  QLabc=[100 90 110]  QCabc=[100 90 110]  Pabcp=[10e3 9e3 11e3]  QLabcp=[100 90 110]  QCabcp=[100 90 110]  Measurements=None  LoadType=constant Z
  load7 : spsThreePhaseSeriesRLCLoadLib/Three-Phase Series RLC Load  LConnTagsString=A|B|C  Configuration=Y (grounded)  NominalVoltage=Vnom_ph_ph  Vabc=[1e3 1e3 1e3]  Vabcp=[1e3 1e3 1e3]  NominalFrequency=60  UnbalancedPower=off  ActivePower=29.05e6  InductivePower=3.10e6  CapacitivePower=0  Pabc=[10e3 9e3 11e3]  QLabc=[100 90 110]  QCabc=[100 90 110]  Pabcp=[10e3 9e3 11e3]  QLabcp=[100 90 110]  QCabcp=[100 90 110]  Measurements=None  LoadType=constant Z
  load8 : spsThreePhaseSeriesRLCLoadLib/Three-Phase Series RLC Load  LConnTagsString=A|B|C  Configuration=Y (grounded)  NominalVoltage=Vnom_ph_ph  Vabc=[1e3 1e3 1e3]  Vabcp=[1e3 1e3 1e3]  NominalFrequency=60  UnbalancedPower=off  ActivePower=190.3e6  InductivePower=81.38e6  CapacitivePower=0  Pabc=[10e3 9e3 11e3]  QLabc=[100 90 110]  QCabc=[100 90 110]  Pabcp=[10e3 9e3 11e3]  QLabcp=[100 90 110]  QCabcp=[100 90 110]  Measurements=None  LoadType=constant Z
  load9 : spsThreePhaseSeriesRLCLoadLib/Three-Phase Series RLC Load  LConnTagsString=A|B|C  Configuration=Y (grounded)  NominalVoltage=Vnom_ph_ph  Vabc=[1e3 1e3 1e3]  Vabcp=[1e3 1e3 1e3]  NominalFrequency=60  UnbalancedPower=off  ActivePower=28.76e6  InductivePower=4.95e6  CapacitivePower=0  Pabc=[10e3 9e3 11e3]  QLabc=[100 90 110]  QCabc=[100 90 110]  Pabcp=[10e3 9e3 11e3]  QLabcp=[100 90 110]  QCabcp=[100 90 110]  Measurements=None  LoadType=constant Z
  powergui : sps_lib/powergui  Priority=1  SimulationMode=Discrete  SampleTime=100e-6  frequency=60  Iterations=50  frequencyindice=50  Pbase=100e3  ErrMax=0.0001  UnitsV=kV  UnitsW=kW  buscounter=0  FunctionMessages=off  echomessages=off  EnableUseOfTLC=off  CurrentSourceSwitches=off  DisableSnubberDevices=off  DisableRonSwitches=off  DisableVfSwitches=off  DisplayEquations=off  AutomaticDiscreteSolvers=off  SolverType=Tustin/Backward Euler (TBE)  Interpol=off  ExternalGateDelay=off  methode=off  Ts=100  x0status=blocks  SPID=off  SwTol=0  HookPort=off  NonlinearTolerance=1e-4  nMaxIteration=100  ContinueOnMaxIteration=off  RestoreLinks=warning  ResistiveCurrentMeasurement=off  Frange=[0:2:500]  Ylog=off  Xlog=on  ShowGrid=off  save=off  variable=ZData  structure=0  ZoomFFT=on  StartTime=0.0  cycles=1  DisplayStyle=1  fundamental=60  FreqAxis=off  MaxFrequency=1000  frequencyindicesteady=1  RmsSteady=1  display=off
  wires:
  Constant3/1 -> NOP2/1
  Constant1/1 -> NOP1/1
  Constant2/1 -> NOP3/1
  Constant4/1 -> Three-Phase Fault/1
  Constant5/1 -> CB2/1
  Constant6/1 -> CB1/1
  Constant7/1 -> CB3/1
  Current Measurement/1 -> Scope/1
  Voltage Measurement/1 -> Scope1/1
  Voltage Measurement1/1 -> Scope3/1
  Current Measurement1/1 -> Scope2/1
  Voltage Measurement2/1 -> Scope5/1
  Current Measurement2/1 -> Scope4/1
  Current Measurement3/1 -> Scope6/1
  Voltage Measurement3/1 -> Scope7/1
  Voltage Measurement4/1 -> Scope9/1
  Current Measurement4/1 -> Scope8/1
  Current Measurement5/1 -> Scope10/1
  Voltage Measurement5/1 -> Scope11/1
  Current Measurement6/1 -> Scope12/1
  Voltage Measurement6/1 -> Scope13/1
  Voltage Measurement7/1 -> Scope15/1
  Current Measurement7/1 -> Scope14/1
  Current Measurement8/1 -> Scope16/1
  Voltage Measurement8/1 -> Scope17/1
  connections:
  14/RConn1 -- Load Flow Bus/LConn1
  14/RConn2 -- Load Flow Bus/LConn2
  14/RConn3 -- Load Flow Bus/LConn3
  13/RConn1 -- Load Flow Bus1/LConn1 -- load13/LConn1
  13/RConn2 -- load13/LConn2 -- Load Flow Bus1/LConn2
  13/RConn3 -- load13/LConn3 -- Load Flow Bus1/LConn3
  L14-13/RConn1 -- 13/LConn1
  L14-13/RConn3 -- 13/LConn3
  L14-13/RConn2 -- 13/LConn2
  12/RConn1 -- Load Flow Bus2/LConn1 -- load12/LConn1
  12/RConn2 -- load12/LConn2 -- Load Flow Bus2/LConn2
  12/RConn3 -- Load Flow Bus2/LConn3 -- load12/LConn3
  L13-12/RConn1 -- 12/LConn1
  L13-12/RConn2 -- 12/LConn2
  L13-12/RConn3 -- 12/LConn3
  11/RConn1 -- load11/LConn1 -- Load Flow Bus3/LConn1
  11/RConn2 -- load11/LConn2 -- Load Flow Bus3/LConn2
  11/RConn3 -- load11/LConn3 -- Load Flow Bus3/LConn3
  L12-11/RConn1 -- 11/LConn1 -- NOP1/LConn1
  L12-11/RConn2 -- 11/LConn2 -- NOP1/LConn2
  11/LConn3 -- L12-11/RConn3 -- NOP1/LConn3
  10/RConn1 -- load10/LConn1 -- Load Flow Bus4/LConn1
  10/RConn2 -- load10/LConn2 -- Load Flow Bus4/LConn2
  10/RConn3 -- load10/LConn3 -- Load Flow Bus4/LConn3
  L11-10/RConn1 -- 10/LConn1
  L11-10/RConn2 -- 10/LConn2
  L11-10/RConn3 -- 10/LConn3
  9/RConn1 -- Load Flow Bus5/LConn1 -- load9/LConn1
  9/RConn2 -- load9/LConn2 -- Load Flow Bus5/LConn2
  9/RConn3 -- load9/LConn3 -- Load Flow Bus5/LConn3
  L10-9/RConn1 -- 9/LConn1
  L10-9/RConn2 -- 9/LConn2
  L10-9/RConn3 -- 9/LConn3
  8/LConn1 -- L9-8/RConn1 -- NOP2/LConn1
  8/LConn2 -- L9-8/RConn2 -- NOP2/LConn2
  8/LConn3 -- L9-8/RConn3 -- NOP2/LConn3
  8/RConn1 -- load8/LConn1 -- Load Flow Bus7/LConn1
  8/RConn2 -- load8/LConn2 -- Load Flow Bus7/LConn2
  8/RConn3 -- Load Flow Bus7/LConn3 -- load8/LConn3
  Three-Phase Transformer (Two Windings)/RConn2 -- 14/LConn2
  Three-Phase Transformer (Two Windings)/RConn3 -- 14/LConn3
  load2/LConn3 -- 2/RConn3 -- Load Flow Bus8/LConn3
  L3-4_2/RConn2 -- 4/LConn2 -- L4-11/RConn2
  Voltage Measurement2/LConn1 -- Current Measurement2/LConn1 -- Voltage Measurement8/LConn1 -- Current Measurement8/LConn1 -- 3/RConn1
  load4/LConn3 -- 4/RConn3 -- Load Flow Bus10/LConn3
  1/RConn1 -- Load Flow Bus6/LConn1
  Three-Phase Transformer (Two Windings)1/RConn3 -- 1/LConn3
  Load Flow Bus12/LConn2 -- 6/RConn2 -- load6/LConn2
  load5/LConn1 -- 5/RConn1 -- Load Flow Bus11/LConn1
  L6-7/RConn3 -- L7-8/RConn3 -- 7/LConn3
  Load Flow Bus9/LConn3 -- 3/RConn3 -- load3/LConn3
  L4-5/RConn3 -- 5/LConn3 -- L5-19/RConn3
  Load Flow Bus12/LConn3 -- 6/RConn3 -- load6/LConn3
  Load Flow Bus12/LConn1 -- 6/RConn1 -- load6/LConn1
  Load Flow Bus11/LConn2 -- 5/RConn2 -- load5/LConn2
  load2/LConn2 -- 2/RConn2 -- Load Flow Bus8/LConn2
  1/RConn2 -- Load Flow Bus6/LConn2
  load3/LConn2 -- 3/RConn2 -- Load Flow Bus9/LConn2
  load4/LConn1 -- 4/RConn1 -- Load Flow Bus10/LConn1
  load2/LConn1 -- Current Measurement/RConn1 -- Load Flow Bus8/LConn1
  1/RConn3 -- Load Flow Bus6/LConn3
  L6-7/RConn2 -- L7-8/RConn2 -- 7/LConn2
  Three-Phase Transformer (Two Windings)1/RConn2 -- 1/LConn2
  load20/LConn1 -- 20/RConn1 -- Load Flow Bus19/LConn1
  Load Flow Bus17/LConn3 -- 18/RConn3 -- load18/LConn3
  Three-Phase Transformer (Two Windings)2/RConn3 -- 15/LConn3
  Load Flow Bus20/LConn2 -- 21/RConn2 -- load21/LConn2
  load19/LConn1 -- 19/RConn1 -- Load Flow Bus18/LConn1
  Load Flow Bus16/LConn3 -- 17/RConn3 -- load17/LConn3
  15/RConn1 -- Load Flow Bus14/LConn1
  Three-Phase Transformer (Two Windings)2/RConn2 -- 15/LConn2
  NOP3/LConn2 -- 19/LConn2 -- L18-19/RConn2
  load18/LConn2 -- 18/RConn2 -- Load Flow Bus17/LConn2
  load16/LConn2 -- 16/RConn2 -- Load Flow Bus15/LConn2
  Load Flow Bus19/LConn3 -- 20/RConn3 -- load20/LConn3
  15/RConn2 -- Load Flow Bus14/LConn2
  load16/LConn3 -- 16/RConn3 -- Load Flow Bus15/LConn3
  15/RConn3 -- Load Flow Bus14/LConn3
  load18/LConn1 -- 18/RConn1 -- Load Flow Bus17/LConn1
  Load Flow Bus19/LConn2 -- 20/RConn2 -- load20/LConn2
  load17/LConn1 -- 17/RConn1 -- Load Flow Bus16/LConn1
  Load Flow Bus20/LConn1 -- 21/RConn1 -- load21/LConn1
  Load Flow Bus20/LConn3 -- 21/RConn3 -- load21/LConn3
  load16/LConn1 -- 16/RConn1 -- Load Flow Bus15/LConn1
  load17/LConn2 -- 17/RConn2 -- Load Flow Bus16/LConn2
  NOP3/LConn3 -- 19/LConn3 -- L18-19/RConn3
  Three-Phase Fault/LConn2 -- L3-4_2/LConn2 -- L3-4_1/RConn2
  Three-Phase Fault/LConn3 -- L3-4_2/LConn3 -- L3-4_1/RConn3
  Three-Phase Fault/LConn1 -- L3-4_2/LConn1 -- L3-4_1/RConn1
  L13-12/LConn1 -- Load Flow Bus1/RConn1
  L13-12/LConn2 -- Load Flow Bus1/RConn2
  L13-12/LConn3 -- Load Flow Bus1/RConn3
  L12-11/LConn1 -- Load Flow Bus2/RConn1
  L12-11/LConn2 -- Load Flow Bus2/RConn2
  L12-11/LConn3 -- Load Flow Bus2/RConn3
  L11-10/LConn2 -- Load Flow Bus3/RConn2
  L11-10/LConn3 -- Load Flow Bus3/RConn3
  L11-10/LConn1 -- Load Flow Bus3/RConn1
  L4-11/LConn1 -- NOP1/RConn1
  L4-11/LConn2 -- NOP1/RConn2
  L4-11/LConn3 -- NOP1/RConn3
  L10-9/LConn1 -- Load Flow Bus4/RConn1
  L10-9/LConn2 -- Load Flow Bus4/RConn2
  L10-9/LConn3 -- Load Flow Bus4/RConn3
  L9-8/LConn1 -- Load Flow Bus5/RConn1
  L9-8/LConn2 -- Load Flow Bus5/RConn2
  L9-8/LConn3 -- Load Flow Bus5/RConn3
  L7-8/LConn1 -- NOP2/RConn1
  L7-8/LConn2 -- NOP2/RConn2
  L7-8/LConn3 -- NOP2/RConn3
  L6-7/LConn1 -- Load Flow Bus12/RConn1
  L6-7/LConn2 -- Load Flow Bus12/RConn2
  L6-7/LConn3 -- Load Flow Bus12/RConn3
  L5-6/LConn1 -- Load Flow Bus11/RConn1
  L5-6/LConn2 -- Load Flow Bus11/RConn2
  L5-6/LConn3 -- Load Flow Bus11/RConn3
  L4-5/LConn1 -- Load Flow Bus10/RConn1
  L4-5/LConn2 -- Load Flow Bus10/RConn2
  L4-5/LConn3 -- Load Flow Bus10/RConn3
  L3-4_1/LConn1 -- Load Flow Bus9/RConn1
  L3-4_1/LConn3 -- Load Flow Bus9/RConn3
  L3-4_1/LConn2 -- Load Flow Bus9/RConn2
  L2-3/LConn1 -- Load Flow Bus8/RConn1
  L2-3/LConn2 -- Load Flow Bus8/RConn2
  L1-2/LConn1 -- Load Flow Bus6/RConn1
  L1-2/LConn2 -- Load Flow Bus6/RConn2
  L1-2/LConn3 -- Load Flow Bus6/RConn3
  L5-19/LConn1 -- NOP3/RConn1
  L5-19/LConn2 -- NOP3/RConn2
  L5-19/LConn3 -- NOP3/RConn3
  L19-20/LConn1 -- Load Flow Bus18/RConn1
  L19-20/LConn2 -- Load Flow Bus18/RConn2
  L19-20/LConn3 -- Load Flow Bus18/RConn3
  L20-21/LConn1 -- Load Flow Bus19/RConn1
  L20-21/LConn2 -- Load Flow Bus19/RConn2
  L20-21/LConn3 -- Load Flow Bus19/RConn3
  L18-19/LConn1 -- Load Flow Bus17/RConn1
  L18-19/LConn2 -- Load Flow Bus17/RConn2
  L18-19/LConn3 -- Load Flow Bus17/RConn3
  L17-18/LConn1 -- Load Flow Bus16/RConn1
  L17-18/LConn2 -- Load Flow Bus16/RConn2
  L17-18/LConn3 -- Load Flow Bus16/RConn3
  L16-17/LConn1 -- Load Flow Bus15/RConn1
  L16-17/LConn2 -- Load Flow Bus15/RConn2
  L16-17/LConn3 -- Load Flow Bus15/RConn3
  L15-16/LConn1 -- Load Flow Bus14/RConn1
  L15-16/LConn2 -- Load Flow Bus14/RConn2
  L15-16/LConn3 -- Load Flow Bus14/RConn3
  L14-13/LConn2 -- Load Flow Bus/RConn2
  L14-13/LConn1 -- Load Flow Bus/RConn1
  L14-13/LConn3 -- Load Flow Bus/RConn3
  CB2/RConn2 -- Three-Phase Transformer (Two Windings)/LConn2
  CB2/RConn1 -- Three-Phase Transformer (Two Windings)/LConn1
  CB2/RConn3 -- Three-Phase Transformer (Two Windings)/LConn3
  CB2/LConn1 -- Load Flow Bus23/RConn1
  CB2/LConn2 -- Load Flow Bus23/RConn2
  Load Flow Bus23/RConn3 -- CB2/LConn3
  Load Flow Bus21/RConn1 -- CB1/LConn1
  Load Flow Bus21/RConn2 -- CB1/LConn2
  Load Flow Bus21/RConn3 -- CB1/LConn3
  CB1/RConn1 -- Three-Phase Transformer (Two Windings)1/LConn1
  CB1/RConn2 -- Three-Phase Transformer (Two Windings)1/LConn2
  CB1/RConn3 -- Three-Phase Transformer (Two Windings)1/LConn3
  Load Flow Bus22/RConn1 -- CB3/LConn1
  Load Flow Bus22/RConn2 -- CB3/LConn2
  CB3/LConn3 -- Load Flow Bus22/RConn3
  CB3/RConn1 -- Three-Phase Transformer (Two Windings)2/LConn1
  CB3/RConn2 -- Three-Phase Transformer (Two Windings)2/LConn2
  CB3/RConn3 -- Three-Phase Transformer (Two Windings)2/LConn3
  L2-3/LConn3 -- Load Flow Bus8/RConn3
  16/LConn1 -- L15-16/RConn1
  16/LConn2 -- L15-16/RConn2
  16/LConn3 -- L15-16/RConn3
  17/LConn1 -- L16-17/RConn1
  17/LConn2 -- L16-17/RConn2
  17/LConn3 -- L16-17/RConn3
  18/LConn1 -- L17-18/RConn1
  18/LConn2 -- L17-18/RConn2
  18/LConn3 -- L17-18/RConn3
  Load Flow Bus18/LConn3 -- 19/RConn3 -- load19/LConn3
  Load Flow Bus18/LConn2 -- 19/RConn2 -- load19/LConn2
  NOP3/LConn1 -- 19/LConn1 -- L18-19/RConn1
  20/LConn1 -- L19-20/RConn1
  20/LConn2 -- L19-20/RConn2
  20/LConn3 -- L19-20/RConn3
  21/LConn1 -- L20-21/RConn1
  21/LConn2 -- L20-21/RConn2
  21/LConn3 -- L20-21/RConn3
  2/LConn1 -- L1-2/RConn1
  2/LConn2 -- L1-2/RConn2
  2/LConn3 -- L1-2/RConn3
  3/LConn1 -- L2-3/RConn1
  3/LConn2 -- L2-3/RConn2
  3/LConn3 -- L2-3/RConn3
  L3-4_2/RConn1 -- 4/LConn1 -- L4-11/RConn1
  load4/LConn2 -- 4/RConn2 -- Load Flow Bus10/LConn2
  L3-4_2/RConn3 -- 4/LConn3 -- L4-11/RConn3
  Load Flow Bus11/LConn3 -- 5/RConn3 -- load5/LConn3
  L4-5/RConn1 -- 5/LConn1 -- L5-19/RConn1
  L4-5/RConn2 -- 5/LConn2 -- L5-19/RConn2
  6/LConn1 -- L5-6/RConn1
  6/LConn2 -- L5-6/RConn2
  6/LConn3 -- L5-6/RConn3
  load7/LConn1 -- Gen7/RConn1 -- 7/RConn1 -- Load Flow Bus13/LConn1
  load7/LConn2 -- Gen7/RConn2 -- 7/RConn2 -- Load Flow Bus13/LConn2
  load7/LConn3 -- Gen7/RConn3 -- 7/RConn3 -- Load Flow Bus13/LConn3
  L6-7/RConn1 -- L7-8/RConn1 -- 7/LConn1
  2/RConn1 -- Voltage Measurement/LConn1 -- Current Measurement/LConn1
  Ground/LConn1 -- Voltage Measurement/LConn2
  Substation1/RConn2 -- Load Flow Bus21/LConn2
  Substation1/RConn3 -- Load Flow Bus21/LConn3
  Ground1/LConn1 -- Voltage Measurement1/LConn2
  Current Measurement1/RConn1 -- Load Flow Bus21/LConn1
  Current Measurement1/LConn1 -- Voltage Measurement1/LConn1 -- Substation1/RConn1
  Ground2/LConn1 -- Voltage Measurement2/LConn2
  Current Measurement2/RConn1 -- Load Flow Bus9/LConn1
  Substation2/RConn2 -- Load Flow Bus23/LConn2
  Substation2/RConn3 -- Load Flow Bus23/LConn3
  Substation3/RConn2 -- Load Flow Bus22/LConn2
  Substation3/RConn3 -- Load Flow Bus22/LConn3
  Ground3/LConn1 -- Voltage Measurement3/LConn2
  Current Measurement3/RConn1 -- Load Flow Bus22/LConn1
  Substation3/RConn1 -- Voltage Measurement3/LConn1 -- Current Measurement3/LConn1
  Ground4/LConn1 -- Voltage Measurement4/LConn2
  Current Measurement4/RConn1 -- 1/LConn1
  Current Measurement4/LConn1 -- Three-Phase Transformer (Two Windings)1/RConn1 -- Voltage Measurement4/LConn1
  Current Measurement5/LConn1 -- Substation2/RConn1 -- Voltage Measurement5/LConn1
  Current Measurement5/RConn1 -- Load Flow Bus23/LConn1
  Ground5/LConn1 -- Voltage Measurement5/LConn2
  Current Measurement6/LConn1 -- Three-Phase Transformer (Two Windings)/RConn1 -- Voltage Measurement6/LConn1
  Current Measurement6/RConn1 -- 14/LConn1
  Ground6/LConn1 -- Voltage Measurement6/LConn2
  Ground7/LConn1 -- Voltage Measurement7/LConn2
  Current Measurement7/RConn1 -- 15/LConn1
  Current Measurement7/LConn1 -- Voltage Measurement7/LConn1 -- Three-Phase Transformer (Two Windings)2/RConn1
  Ground8/LConn1 -- Voltage Measurement8/LConn2
  Current Measurement8/RConn1 -- load3/LConn1

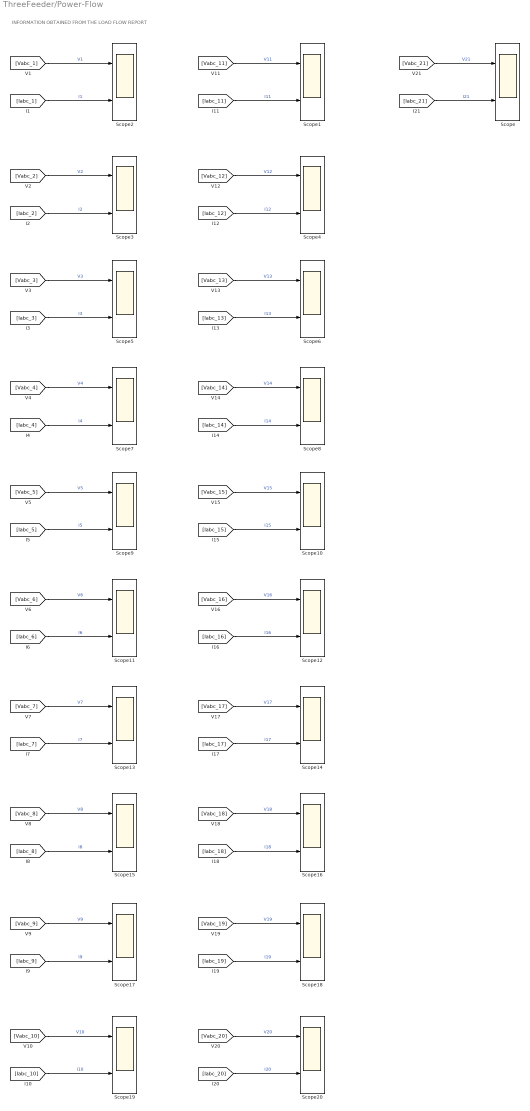
== system ThreeFeeder/Power-Flow ==
  note: INFORMATION OBTAINED FROM THE LOAD FLOW REPORT
  Scope{,1..20} (21 alike) : Scope  NumInputPorts=2
  wires:
  [Vabc_1] -> Scope2/1  "V1"
  [Iabc_1] -> Scope2/2  "I1"
  [Iabc_2] -> Scope3/2  "I2"
  [Vabc_2] -> Scope3/1  "V2"
  [Iabc_3] -> Scope5/2  "I3"
  [Vabc_3] -> Scope5/1  "V3"
  [Iabc_4] -> Scope7/2  "I4"
  [Vabc_4] -> Scope7/1  "V4"
  [Iabc_5] -> Scope9/2  "I5"
  [Vabc_5] -> Scope9/1  "V5"
  [Iabc_6] -> Scope11/2  "I6"
  [Vabc_6] -> Scope11/1  "V6"
  [Iabc_7] -> Scope13/2  "I7"
  [Vabc_7] -> Scope13/1  "V7"
  [Iabc_8] -> Scope15/2  "I8"
  [Vabc_8] -> Scope15/1  "V8"
  [Iabc_9] -> Scope17/2  "I9"
  [Vabc_9] -> Scope17/1  "V9"
  [Iabc_10] -> Scope19/2  "I10"
  [Vabc_10] -> Scope19/1  "V10"
  [Iabc_11] -> Scope1/2  "I11"
  [Vabc_11] -> Scope1/1  "V11"
  [Iabc_12] -> Scope4/2  "I12"
  [Vabc_12] -> Scope4/1  "V12"
  [Iabc_13] -> Scope6/2  "I13"
  [Vabc_13] -> Scope6/1  "V13"
  [Iabc_14] -> Scope8/2  "I14"
  [Vabc_14] -> Scope8/1  "V14"
  [Iabc_15] -> Scope10/2  "I15"
  [Vabc_15] -> Scope10/1  "V15"
  [Iabc_16] -> Scope12/2  "I16"
  [Vabc_16] -> Scope12/1  "V16"
  [Iabc_17] -> Scope14/2  "I17"
  [Vabc_17] -> Scope14/1  "V17"
  [Iabc_18] -> Scope16/2  "I18"
  [Vabc_18] -> Scope16/1  "V18"
  [Iabc_19] -> Scope18/2  "I19"
  [Vabc_19] -> Scope18/1  "V19"
  [Iabc_20] -> Scope20/2  "I20"
  [Vabc_20] -> Scope20/1  "V20"
  [Iabc_21] -> Scope/2  "I21"
  [Vabc_21] -> Scope/1  "V21"

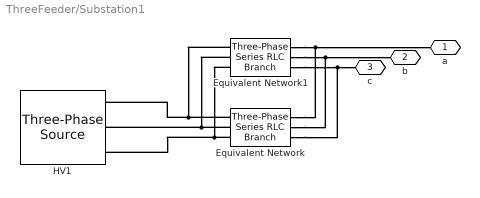
== system ThreeFeeder/Substation1 ==
  Equivalent Network : spsThreePhaseSeriesRLCBranchLib/Three-Phase Series RLC Branch  LConnTagsString=A|B|C  RConnTagsString=A|B|C  BranchType=RL  Resistance=5  Inductance=1  Capacitance=1.0  Measurements=None
  Equivalent Network1 : spsThreePhaseSeriesRLCBranchLib/Three-Phase Series RLC Branch  LConnTagsString=A|B|C  RConnTagsString=A|B|C  BranchType=C  Resistance=5  Inductance=1  Capacitance=1  Measurements=None
  HV1 : spsThreePhaseSourceLib/Three-Phase Source  InternalConnection=Yg  VoltagePhases=off  Voltage=115e3  PhaseAngle=0  Voltage_phases=[1 1 1]*(115e3)/sqrt(3)  PhaseAngles_phases=[0 -120 +120]  Frequency=Frequency  NonIdealSource=off  SpecifyImpedance=on  Resistance=0.8929  Inductance=16.58e-3  ShortCircuitLevel=Apparent_power_gen1  BaseVoltage=Vnom_ph_ph  XRratio=8  BusType=swing  Pref=1000e6  Qref=0  Prefabc=[10e3, 10e3, 10e3]  Qrefabc=[0, 0, 0]  Qmin=[-1500 -1500 -1500]*1e6  Qmax=[1500 1500 1500]*1e6
  a : PMIOPort  Side=Right
  b : PMIOPort  Port=2  Side=Right
  c : PMIOPort  Port=3  Side=Right
  connections:
  Equivalent Network/LConn2 -- Equivalent Network1/LConn2 -- HV1/RConn2
  Equivalent Network1/RConn3 -- Equivalent Network/RConn3 -- c/RConn1
  Equivalent Network/LConn3 -- Equivalent Network1/LConn3 -- HV1/RConn3
  Equivalent Network/LConn1 -- Equivalent Network1/LConn1 -- HV1/RConn1
  Equivalent Network1/RConn1 -- Equivalent Network/RConn1 -- a/RConn1
  Equivalent Network1/RConn2 -- Equivalent Network/RConn2 -- b/RConn1

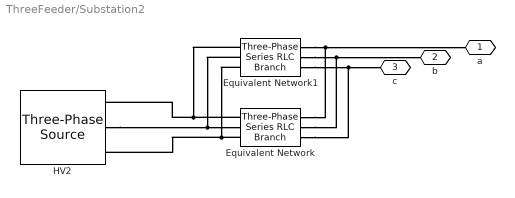
== system ThreeFeeder/Substation2 ==
  Equivalent Network : spsThreePhaseSeriesRLCBranchLib/Three-Phase Series RLC Branch  LConnTagsString=A|B|C  RConnTagsString=A|B|C  BranchType=RL  Resistance=5  Inductance=1  Capacitance=1.0  Measurements=None
  Equivalent Network1 : spsThreePhaseSeriesRLCBranchLib/Three-Phase Series RLC Branch  LConnTagsString=A|B|C  RConnTagsString=A|B|C  BranchType=C  Resistance=5  Inductance=1  Capacitance=1  Measurements=None
  HV2 : spsThreePhaseSourceLib/Three-Phase Source  InternalConnection=Yg  VoltagePhases=off  Voltage=115e3  PhaseAngle=0  Voltage_phases=[1 1 1]*(115e3)/sqrt(3)  PhaseAngles_phases=[0 -120 +120]  Frequency=Frequency  NonIdealSource=off  SpecifyImpedance=on  Resistance=0.8929  Inductance=16.58e-3  ShortCircuitLevel=Apparent_power_gen1  BaseVoltage=Vnom_ph_ph  XRratio=8  BusType=PV  Pref=1000e6  Qref=0  Prefabc=[10e3, 10e3, 10e3]  Qrefabc=[0, 0, 0]  Qmin=[-1500 -1500 -1500]*1e6  Qmax=[1500 1500 1500]*1e6
  a : PMIOPort  Side=Right
  b : PMIOPort  Port=2  Side=Right
  c : PMIOPort  Port=3  Side=Right
  connections:
  Equivalent Network/LConn1 -- Equivalent Network1/LConn1 -- HV2/RConn1
  Equivalent Network1/RConn1 -- Equivalent Network/RConn1 -- a/RConn1
  Equivalent Network1/RConn2 -- Equivalent Network/RConn2 -- b/RConn1
  Equivalent Network1/RConn3 -- Equivalent Network/RConn3 -- c/RConn1
  Equivalent Network/LConn3 -- Equivalent Network1/LConn3 -- HV2/RConn3
  HV2/RConn2 -- Equivalent Network1/LConn2 -- Equivalent Network/LConn2
